simulink model "pi_controller_demo"  (R2018a)
settings: Solver=VariableStepAuto  StartTime=0.0  StopTime=10.0  FixedStep=0.001  RelTol=1e-3
libraries: simulink x1
settings Model: Creator=taoyi  LastModifiedBy=taoyi

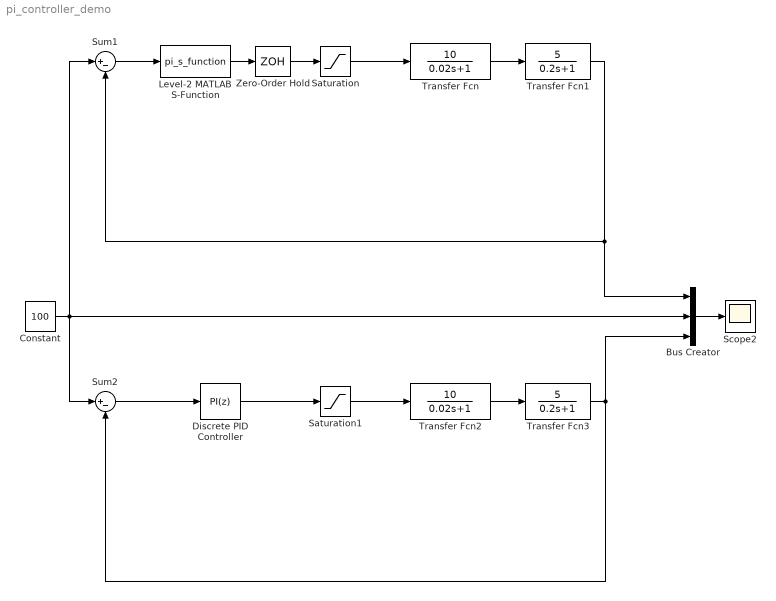
== system pi_controller_demo ==
  Bus Creator : BusCreator  Inputs=3
  Constant : Constant  Value=100
  Discrete PID Controller : simulink/Continuous/PID Controller  Controller=PI  TimeDomain=Discrete-time  SampleTime=0.005  IntegratorMethod=Forward Euler  FilterMethod=Forward Euler  Form=Parallel  UseFilter=on  ControllerParametersSource=internal  P=0.1  I=1  D=0  N=100  InitialConditionSource=internal  InitialConditionForIntegrator=0  InitialConditionForFilter=0  ExternalReset=none  LimitOutput=off  UpperSaturationLimit=inf  LowerSaturationLimit=-inf  LinearizeAsGain=off  AntiWindupMode=none  Kb=1  TrackingMode=off  Kt=1  PParamMin=[]  PParamMax=[]  IParamMin=[]  IParamMax=[]  DParamMin=[]  DParamMax=[]  NParamMin=[]  NParamMax=[]  KbParamMin=[]  KbParamMax=[]  KtParamMin=[]  KtParamMax=[]  POutMin=[]  POutMax=[]  IOutMin=[]  IOutMax=[]  DOutMin=[]  DOutMax=[]  NOutMin=[]  NOutMax=[]  KbOutMin=[]  KbOutMax=[]  KtOutMin=[]  KtOutMax=[]  IntegratorOutMin=[]  IntegratorOutMax=[]  FilterOutMin=[]  FilterOutMax=[]  SumOutMin=[]  SumOutMax=[]  SumI1OutMin=[]  SumI1OutMax=[]  SumI2OutMin=[]  SumI2OutMax=[]  SumI3OutMin=[]  SumI3OutMax=[]  SumDOutMin=[]  SumDOutMax=[]  SaturationOutMin=[]  SaturationOutMax=[]  IntegratorContinuousStateAttributes=''  IntegratorStateMustResolveToSignalObject=off  IntegratorRTWStateStorageClass=Auto  FilterContinuousStateAttributes=''  FilterStateMustResolveToSignalObject=off  FilterRTWStateStorageClass=Auto  DifferentiatorICPrevScaledInput=0  DifferentiatorOutMin=[]  DifferentiatorOutMax=[]  FilterDiffOutCoefMin=[]  FilterDiffOutCoefMax=[]  SumDenOutMin=[]  SumDenOutMax=[]  SumNumOutMin=[]  SumNumOutMax=[]  ReciprocalOutMin=[]  ReciprocalOutMax=[]  DivideOutMin=[]  DivideOutMax=[]  TunerSelectOption=Transfer Function Based (PID Tuner App)
  Level-2 MATLAB S-Function : M-S-Function  FunctionName=pi_s_function
  Saturation : Saturate  UpperLimit=10  LowerLimit=-10
  Saturation1 : Saturate  UpperLimit=10  LowerLimit=-10
  Scope2 : Scope
  Sum1 : Sum  Inputs=|+-
  Sum2 : Sum  Inputs=|+-
  Transfer Fcn : TransferFcn  Numerator=[10]  Denominator=[0.02 1]
  Transfer Fcn1 : TransferFcn  Numerator=[5]  Denominator=[0.2 1]
  Transfer Fcn2 : TransferFcn  Numerator=[10]  Denominator=[0.02 1]
  Transfer Fcn3 : TransferFcn  Numerator=[5]  Denominator=[0.2 1]
  Zero-Order Hold : ZeroOrderHold  SampleTime=-1
  wires:
  Bus Creator/1 -> Scope2/1
  Transfer Fcn2/1 -> Transfer Fcn3/1
  Transfer Fcn3/1 -> Sum2/2, Bus Creator/3
  Saturation1/1 -> Transfer Fcn2/1
  Saturation/1 -> Transfer Fcn/1
  Transfer Fcn1/1 -> Sum1/2, Bus Creator/1
  Constant/1 -> Sum1/1, Sum2/1, Bus Creator/2
  Transfer Fcn/1 -> Transfer Fcn1/1
  Level-2 MATLAB S-Function/1 -> Zero-Order Hold/1
  Zero-Order Hold/1 -> Saturation/1
  Sum1/1 -> Level-2 MATLAB S-Function/1
  Sum2/1 -> Discrete PID Controller/1
  Discrete PID Controller/1 -> Saturation1/1
